simulink model "Idq_core_control"  (R2023b)
settings: configuration reference "ctrl_tsk_conf" (kept outside this file)
libraries: simulink x1
settings Model: DataDictionary=fmuGenerationDictionay.sldd  Creator=Veimar  LastModifiedBy=Veimar
settings ConfigSetRef: SourceName=ctrl_tsk_conf

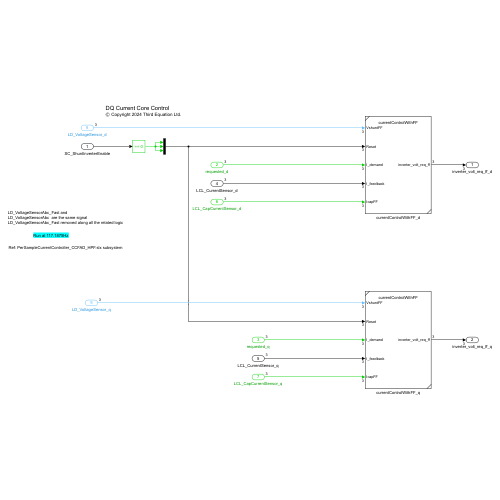
[thumbnail: Simulink's stored preview of the top-level diagram]
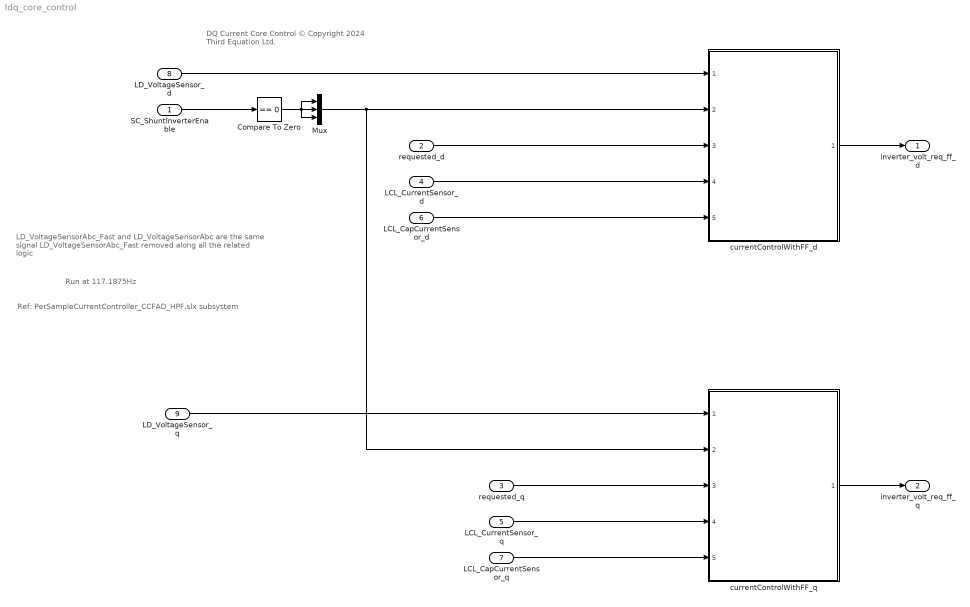
== system Idq_core_control ==
  note: Ref: PerSampleCurrentController_CCFAD_HPF.slx subsystem
  note: DQ Current Core Control
      | © Copyright 2024 Third Equation Ltd.
  note: LD_VoltageSensorAbc_Fast and
      | LD_VoltageSensorAbc  are the same signal
      | LD_VoltageSensorAbc_Fast removed along all the related logic
  note: Run at 117.1875Hz
  SC_ShuntInverterEnable : Inport  OutDataTypeStr=boolean  PortDimensions=1
  requested_d : Inport  Port=2  OutDataTypeStr=single  PortDimensions=3
  requested_q : Inport  Port=3  OutDataTypeStr=single  PortDimensions=3
  LCL_CurrentSensor_d : Inport  Port=4  OutDataTypeStr=single  PortDimensions=3
  LCL_CurrentSensor_q : Inport  Port=5  OutDataTypeStr=single  PortDimensions=3
  LCL_CapCurrentSensor_d : Inport  Port=6  OutDataTypeStr=single  PortDimensions=3
  LCL_CapCurrentSensor_q : Inport  Port=7  OutDataTypeStr=single  PortDimensions=3
  LD_VoltageSensor_d : Inport  Port=8  OutDataTypeStr=single  PortDimensions=3
  LD_VoltageSensor_q : Inport  Port=9  OutDataTypeStr=single  PortDimensions=3
  Compare To Zero : simulink/Logic and Bit Operations/Compare To Zero  relop===  OutDataTypeStr=boolean
  Mux : Mux  Inputs=3
  currentControlWithFF_d : Subsystem  ReferencedSubsystem=currentControlWithFF
      settings: PermitHierarchicalResolution=None
  currentControlWithFF_q : Subsystem  ReferencedSubsystem=currentControlWithFF
      settings: PermitHierarchicalResolution=None
  inverter_volt_req_ff_d : Outport  OutDataTypeStr=single  PortDimensions=3
  inverter_volt_req_ff_q : Outport  Port=2  OutDataTypeStr=single  PortDimensions=3
  wires:
  LD_VoltageSensor_q/1 -> currentControlWithFF_q/1
  Compare To Zero/1 -> Mux/3, Mux/1, Mux/2
  LD_VoltageSensor_d/1 -> currentControlWithFF_d/1
  Mux/1 -> currentControlWithFF_q/2, currentControlWithFF_d/2
  LCL_CapCurrentSensor_q/1 -> currentControlWithFF_q/5
  currentControlWithFF_q/1 -> inverter_volt_req_ff_q/1
  LCL_CurrentSensor_d/1 -> currentControlWithFF_d/4
  currentControlWithFF_d/1 -> inverter_volt_req_ff_d/1
  requested_d/1 -> currentControlWithFF_d/3
  SC_ShuntInverterEnable/1 -> Compare To Zero/1
  LCL_CapCurrentSensor_d/1 -> currentControlWithFF_d/5
  requested_q/1 -> currentControlWithFF_q/3
  LCL_CurrentSensor_q/1 -> currentControlWithFF_q/4
